simulink model "twsbr_cascade_pid"  (R2026a)
settings: Solver=ode45  StopTime=8.0  MaxStep=0.001  RelTol=1e-9  AbsTol=1e-11
model workspace (MAT data in the model file):
  controller_reset_data = [0  1; 0.001  0; 8  0]
  disturbance_force_data = [0  0; 8  0]
  disturbance_torque_data = [0  0; 8  0]
  position_reference_data = [0  0; 8  0]
settings Model: Creator=Linxiuqi  LastModifiedBy=Linxiuqi

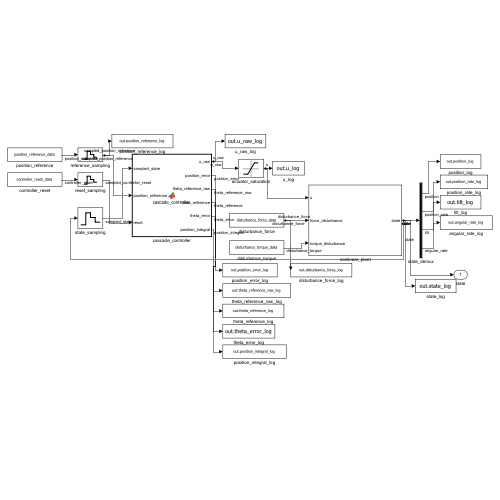
[thumbnail: Simulink's stored preview of the top-level diagram]
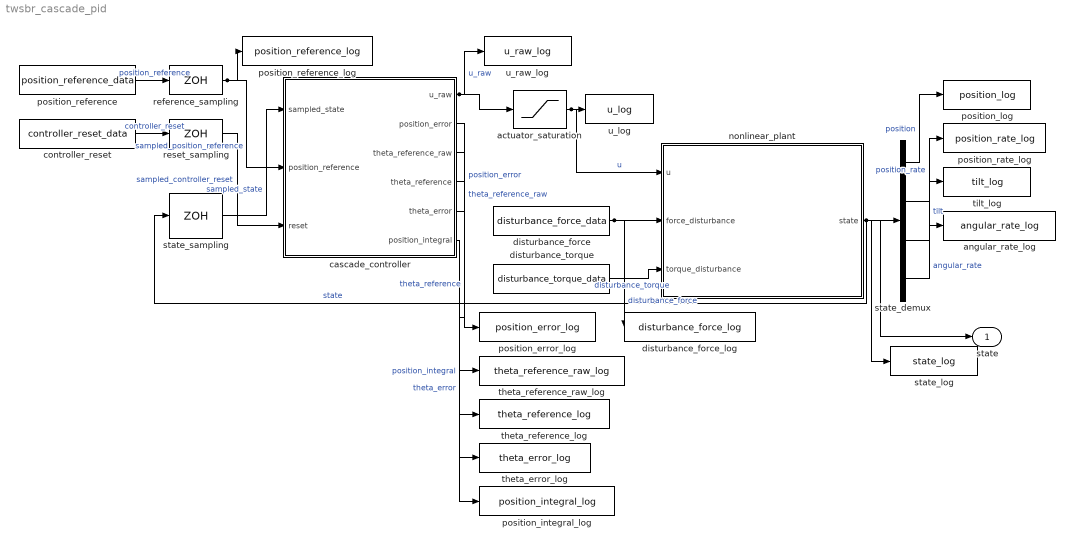
== system twsbr_cascade_pid ==
  actuator_saturation : Saturate  UpperLimit=1  LowerLimit=-1
  angular_rate_log : ToWorkspace  VariableName=angular_rate_log  SaveFormat=Structure With Time  SampleTime=-1
  cascade_controller : MATLAB Function  TreatAsAtomicUnit=on
  controller_reset : FromWorkspace  VariableName=controller_reset_data  Interpolate=off  OutputAfterFinalValue=Holding final value
  disturbance_force : FromWorkspace  VariableName=disturbance_force_data  Interpolate=off  OutputAfterFinalValue=Holding final value
  disturbance_force_log : ToWorkspace  VariableName=disturbance_force_log  SaveFormat=Structure With Time  SampleTime=-1
  disturbance_torque : FromWorkspace  VariableName=disturbance_torque_data  Interpolate=off  OutputAfterFinalValue=Holding final value
  nonlinear_plant : Subsystem
  position_error_log : ToWorkspace  VariableName=position_error_log  SaveFormat=Structure With Time  SampleTime=-1
  position_integral_log : ToWorkspace  VariableName=position_integral_log  SaveFormat=Structure With Time  SampleTime=-1
  position_log : ToWorkspace  VariableName=position_log  SaveFormat=Structure With Time  SampleTime=-1
  position_rate_log : ToWorkspace  VariableName=position_rate_log  SaveFormat=Structure With Time  SampleTime=-1
  position_reference : FromWorkspace  VariableName=position_reference_data  Interpolate=off  OutputAfterFinalValue=Holding final value
  position_reference_log : ToWorkspace  VariableName=position_reference_log  SaveFormat=Structure With Time  SampleTime=-1
  reference_sampling : ZeroOrderHold  SampleTime=0.01
  reset_sampling : ZeroOrderHold  SampleTime=0.01
  state_demux : Demux
  state_log : ToWorkspace  VariableName=state_log  SaveFormat=Structure With Time  SampleTime=-1
  state_sampling : ZeroOrderHold  SampleTime=0.01
  theta_error_log : ToWorkspace  VariableName=theta_error_log  SaveFormat=Structure With Time  SampleTime=-1
  theta_reference_log : ToWorkspace  VariableName=theta_reference_log  SaveFormat=Structure With Time  SampleTime=-1
  theta_reference_raw_log : ToWorkspace  VariableName=theta_reference_raw_log  SaveFormat=Structure With Time  SampleTime=-1
  tilt_log : ToWorkspace  VariableName=tilt_log  SaveFormat=Structure With Time  SampleTime=-1
  u_log : ToWorkspace  VariableName=u_log  SaveFormat=Structure With Time  SampleTime=-1
  u_raw_log : ToWorkspace  VariableName=u_raw_log  SaveFormat=Structure With Time  SampleTime=-1
  state : Outport
  wires:
  position_reference/1 -> reference_sampling/1  "position_reference"
  reference_sampling/1 -> cascade_controller/2(position_reference), position_reference_log/1  "sampled_position_reference"
  controller_reset/1 -> reset_sampling/1  "controller_reset"
  reset_sampling/1 -> cascade_controller/3(reset)  "sampled_controller_reset"
  nonlinear_plant/1(state) -> state_sampling/1, state_demux/1, state/1, state_log/1  "state"
  state_sampling/1 -> cascade_controller/1(sampled_state)  "sampled_state"
  cascade_controller/1(u_raw) -> actuator_saturation/1, u_raw_log/1  "u_raw"
  cascade_controller/2(position_error) -> position_error_log/1  "position_error"
  cascade_controller/3(theta_reference_raw) -> theta_reference_raw_log/1  "theta_reference_raw"
  cascade_controller/4(theta_reference) -> theta_reference_log/1  "theta_reference"
  cascade_controller/5(theta_error) -> theta_error_log/1  "theta_error"
  cascade_controller/6(position_integral) -> position_integral_log/1  "position_integral"
  actuator_saturation/1 -> nonlinear_plant/1(u), u_log/1  "u"
  disturbance_force/1 -> nonlinear_plant/2(force_disturbance), disturbance_force_log/1  "disturbance_force"
  disturbance_torque/1 -> nonlinear_plant/3(torque_disturbance)  "disturbance_torque"
  state_demux/1 -> position_log/1  "position"
  state_demux/2 -> position_rate_log/1  "position_rate"
  state_demux/3 -> tilt_log/1  "tilt"
  state_demux/4 -> angular_rate_log/1  "angular_rate"

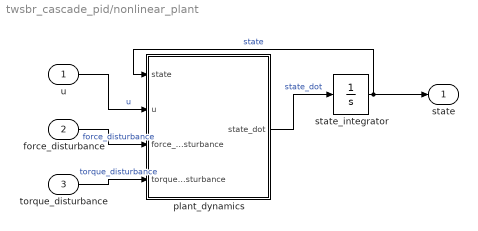
== system twsbr_cascade_pid/nonlinear_plant ==
  u : Inport
  force_disturbance : Inport  Port=2
  torque_disturbance : Inport  Port=3
  plant_dynamics : MATLAB Function  TreatAsAtomicUnit=on
  state_integrator : Integrator  InitialCondition=[0;0;0;0]
  state : Outport
  wires:
  plant_dynamics/1(state_dot) -> state_integrator/1  "state_dot"
  torque_disturbance/1 -> plant_dynamics/4(torque_disturbance)  "torque_disturbance"
  force_disturbance/1 -> plant_dynamics/3(force_disturbance)  "force_disturbance"
  u/1 -> plant_dynamics/2(u)  "u"
  state_integrator/1 -> state/1, plant_dynamics/1(state)  "state"

== matlab function twsbr_cascade_pid/nonlinear_plant/plant_dynamics ==
  data: state input; u input; state_dot output; force_disturbance input; torque_disturbance input
function state_dot = plant_dynamics(state, u, force_disturbance, torque_disturbance)
%#codegen
body_mass = 1.2;
wheel_mass = 0.29999999999999999;
com_length = 0.17999999999999999;
body_inertia = 0.025000000000000001;
damping = 0.050000000000000003;
gravity = 9.8100000000000005;
motor_gain = 12;
x_dot = state(2);
theta = state(3);
theta_dot = state(4);
force = motor_gain * u + force_disturbance;
mass_sum = wheel_mass + body_mass;
rotational_term = body_inertia + body_mass * com_length^2;
coupling = body_mass * com_length * cos(theta);
rhs_position = force - damping * x_dot + body_mass * com_length * theta_dot^2 * sin(theta);
rhs_angle = body_mass * gravity * com_length * sin(theta) + torque_disturbance;
determinant = mass_sum * rotational_term - coupling^2;
x_ddot = (rotational_term * rhs_position - coupling * rhs_angle) / determinant;
theta_ddot = (-coupling * rhs_position + mass_sum * rhs_angle) / determinant;
state_dot = [x_dot; x_ddot; theta_dot; theta_ddot];
end

== matlab function twsbr_cascade_pid/cascade_controller ==
  data: sampled_state input; u_raw output; position_reference input; reset input; position_error output; theta_reference_raw output; theta_reference output; theta_error output; position_integral output
function [u_raw, position_error, theta_reference_raw, theta_reference, theta_error, position_integral] = cascade_controller(sampled_state, position_reference, reset)
%#codegen
persistent position_integral_state
if isempty(position_integral_state) || reset ~= 0
    position_integral_state = 0.0;
end
kp_x = 0.24100028146267993;
ki_x = 0.00039620677559885719;
kd_x = 0.1930824033173246;
kp_theta = 9.2549291491775563;
kd_theta = 1.0113335430173094;
sample_time = 0.01;
theta_reference_limit = 0.20943951023931956;
position_integral_limit = 1000000;
x = sampled_state(1);
x_dot = sampled_state(2);
theta = sampled_state(3);
theta_dot = sampled_state(4);
position_integral = position_integral_state;
position_error = position_reference - x;
theta_reference_raw = kp_x * position_error + ki_x * position_integral - kd_x * x_dot;
theta_reference = min(max(theta_reference_raw, -theta_reference_limit), theta_reference_limit);
theta_error = theta - theta_reference;
u_raw = kp_theta * theta_error + kd_theta * theta_dot;
position_integral_state = position_integral_state + sample_time * position_error;
position_integral_state = min(max(position_integral_state, -position_integral_limit), position_integral_limit);
end
